simulink model "Mdl_Speed"  (R2024b)
settings: Solver=FixedStepDiscrete  StartTime=0.0  StopTime=10.0  FixedStep=0.1  RelTol=1e-3  EnableMultiTasking=on
values from neighbouring files (symbols this model uses):
  AI_TEMP_ADC_COUNT_1586 = mpt.Parameter    [Mdl_Speed_lookup.m]
  AI_TEMP_ADC_COUNT_1727 = mpt.Parameter    [Mdl_Speed_lookup.m]
  AI_TEMP_ADC_COUNT_1792 = mpt.Parameter    [Mdl_Speed_lookup.m]
  AI_TEMP_ADC_COUNT_1891 = mpt.Parameter    [Mdl_Speed_lookup.m]
  C_ADR = mpt.Parameter    [Mdl_Speed_lookup.m]
  C_CANADA = mpt.Parameter    [Mdl_Speed_lookup.m]
  C_EUROPE = mpt.Parameter    [Mdl_Speed_lookup.m]
  C_KOREA = mpt.Parameter    [Mdl_Speed_lookup.m]
  C_MEXICO = mpt.Parameter    [Mdl_Speed_lookup.m]
  C_UK = mpt.Parameter    [Mdl_Speed_lookup.m]
  C_USA = mpt.Parameter    [Mdl_Speed_lookup.m]
  eSP_ADR = mpt.Parameter    [Speed_Table_Type_param.m]
  eSP_CANADA = mpt.Parameter    [Speed_Table_Type_param.m]
  eSP_ECE = mpt.Parameter    [Speed_Table_Type_param.m]
  eSP_EUROPE = mpt.Parameter    [Speed_Table_Type_param.m]
  eSP_KOREA_FMVSS = mpt.Parameter    [Speed_Table_Type_param.m]
  eSP_KOREA_UN_R = mpt.Parameter    [Speed_Table_Type_param.m]
  eSP_MEXICO_FMVSS = mpt.Parameter    [Speed_Table_Type_param.m]
  eSP_MEXICO_UN_R = mpt.Parameter    [Speed_Table_Type_param.m]
  eSP_UK = mpt.Parameter    [Speed_Table_Type_param.m]
  eSP_USA = mpt.Parameter    [Speed_Table_Type_param.m]
  INDEX_MCUID0262 = mpt.Parameter    [Mdl_Speed_lookup.m]
  INDEX_MCUID0263 = mpt.Parameter    [Mdl_Speed_lookup.m]
  Initial_data = mpt.Parameter    [Mdl_Speed_lookup.m]
  MCUID0809 = mpt.Parameter    [Mdl_Speed_DD.m]
  MCUID0810 = mpt.Parameter    [Mdl_Speed_DD.m]
  MCUID_MAX_VAL = mpt.Parameter    [Mdl_Speed_lookup.m]
  MIN_SPEED_VALUE = mpt.Parameter    [Mdl_Speed_lookup.m]
  RESOLUTION_VAL_100 = mpt.Parameter    [Mdl_Speed_lookup.m]
  RESOLUTION_VAL_103 = mpt.Parameter    [Mdl_Speed_lookup.m]
  RESOLUTION_VAL_50 = mpt.Parameter    [Mdl_Speed_lookup.m]
  RESOLUTION_VAL_64 = mpt.Parameter    [Mdl_Speed_lookup.m]
  RESOLUTION_VAL_MINUS_100 = mpt.Parameter    [Mdl_Speed_lookup.m]
  SPEED_AVG_REF = mpt.Parameter    [Mdl_Speed_lookup.m]
  SPEED_CHECK_VALUE_ONE = mpt.Parameter    [Mdl_Speed_lookup.m]
  SPEED_UPDATE_0_28S = mpt.Parameter    [Mdl_Speed_lookup.m]
  SPEED_UPDATE_0_5S = mpt.Parameter    [Mdl_Speed_lookup.m]
  SPEED_UPDATE_1_5S = mpt.Parameter    [Mdl_Speed_lookup.m]
  SPEED_UPDATE_1S = mpt.Parameter    [Mdl_Speed_lookup.m]
  SPEED_ZERO = mpt.Parameter    [Mdl_Speed_lookup.m]
  VAL_ONE = mpt.Parameter    [Mdl_Speed_lookup.m]
  VAL_ZERO = mpt.Parameter    [Mdl_Speed_lookup.m]
undefined symbols (not defined in the file or in its folder): Arr_u8_100_type_instance, Arr_u8_1024_type_instance, Arr_u8_10_type_instance, Arr_u8_128_type_instance, Arr_u8_16_type_instance, Arr_u8_17_type_instance, Arr_u8_2048_type_instance, Arr_u8_256_type_instance, Arr_u8_32_type_instance, Arr_u8_3_type_instance, Arr_u8_46_type_instance, Arr_u8_48_type_instance, Arr_u8_61_type_instance, Arr_u8_64_type_instance, Arr_u8_8_type_instance, Arr_u8_9_type_instance, CLUSTER_ACTIVE, eIO_ADC_AI_TEMP_RTC, eSIGNAL_MISSING, eSIGNAL_NEVER_RECEIVED, eVehicleSpeedABSIn, IgnOff, IgnOn, IoHwAb_AdcSignalIdType_type_instance, IoHwAb_ErrorType_type_instance, pJustRcvdStatus, RxCan_SignalClearJustRcvdStatus, RxCan_SignalGetJustRcvdStatus, RxCan_SignalInvalidProcessingControl, RxCan_SignalMissingProcessingControl, RxCan_SignalNRProcessingControl, SignalId, SPEED_MAX_RESOLUTION, Status, tRxSignalId_type_instance, tRxSignalJustRcvdStatus_type_instance, tRxSignalStatus_type_instance
libraries: simulink x9
(part 3 of 3)

== system Mdl_Speed/Mdl_Speed_Task_sys/Digital_speed/Subsystem1/Interpolation&Trim_data/Subsystem/Speed_trimming_KM ==
  speed_avg : Inport  OutDataTypeStr=uint16
  Constant : Constant  Value=RESOLUTION_VAL_100  OutDataTypeStr=uint16
  Constant2 : Constant  Value=RESOLUTION_VAL_100
  Divide : Product  Inputs=*/  SaturateOnIntegerOverflow=on
  If : If  IfExpression=u1 < 50
  Merge : Merge
  Mod : Math  Operator=mod  SignedPower=on
  Speed_trim_Less_than_0.5 : Subsystem  TreatAsAtomicUnit=on
  Speed_trim_greater_than_equal_to_0.5 : Subsystem  TreatAsAtomicUnit=on
  Speed_trim : Outport  VectorParamsAs1DForOutWhenUnconnected=off
  wires:
  [Speed_avg] -> Divide/1
  Constant2/1 -> Divide/2
  If/1 -> Speed_trim_Less_than_0.5/Action
  Divide/1 -> Speed_trim_greater_than_equal_to_0.5/1(Speed_avg), Speed_trim_Less_than_0.5/1(Speed_avg)
  Speed_trim_Less_than_0.5/1(Speed_trim) -> Merge/1
  Speed_trim_greater_than_equal_to_0.5/1(Speed_trim) -> Merge/2
  If/2 -> Speed_trim_greater_than_equal_to_0.5/Action
  Mod/1 -> If/1
  [Speed_avg] -> Mod/1
  Constant/1 -> Mod/2
  Merge/1 -> Speed_trim/1
  speed_avg/1 -> [Speed_avg]

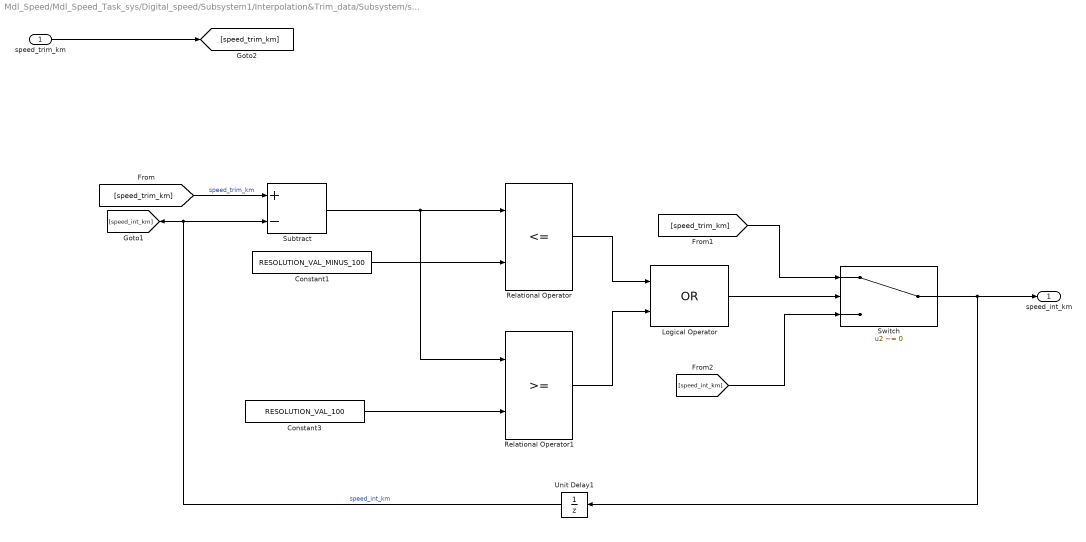
== system Mdl_Speed/Mdl_Speed_Task_sys/Digital_speed/Subsystem1/Interpolation&Trim_data/Subsystem/speed_internal_km ==
  speed_trim_km : Inport
  Constant1 : Constant  Value=RESOLUTION_VAL_MINUS_100  OutDataTypeStr=int8
  Constant3 : Constant  Value=RESOLUTION_VAL_100  OutDataTypeStr=uint16
  Logical Operator : Logic  Operator=OR  AllPortsSameDT=off  OutDataTypeStr=boolean
  Relational Operator : RelationalOperator  Operator=<=  OutDataTypeStr=boolean  RndMeth=Simplest  InputSameDT=off
  Relational Operator1 : RelationalOperator  OutDataTypeStr=boolean  RndMeth=Simplest  InputSameDT=off
  Subtract : Sum  Inputs=+-  OutDataTypeStr=int32
  Switch : Switch  Criteria=u2 ~= 0  SaturateOnIntegerOverflow=off  InputSameDT=off
  Unit Delay1 : UnitDelay  SampleTime=-1  StateName=Prev_speed_Int_km  HasFrameUpgradeWarning=on
  speed_int_km : Outport  VectorParamsAs1DForOutWhenUnconnected=off
  wires:
  [speed_trim_km] -> Subtract/1  "speed_trim_km"
  Unit Delay1/1 -> [speed_int_km], Subtract/2  "speed_int_km"
  Subtract/1 -> Relational Operator1/1, Relational Operator/1
  Constant1/1 -> Relational Operator/2
  Constant3/1 -> Relational Operator1/2
  Relational Operator/1 -> Logical Operator/1
  Relational Operator1/1 -> Logical Operator/2
  Logical Operator/1 -> Switch/2
  [speed_trim_km] -> Switch/1
  speed_trim_km/1 -> [speed_trim_km]
  Switch/1 -> speed_int_km/1, Unit Delay1/1
  [speed_int_km] -> Switch/3

== system Mdl_Speed/Mdl_Speed_Task_sys/Digital_speed/Subsystem1/Interpolation&Trim_data/Subsystem1/Speed_target_Miles ==
  Speed_int : Inport
  Constant2 : Constant  Value=RESOLUTION_VAL_100  OutDataTypeStr=uint16
  Constant3 : Constant  Value=RESOLUTION_VAL_100  OutDataTypeStr=uint16
  Divide : Product  Inputs=*/  SaturateOnIntegerOverflow=on
  If : If  IfExpression=u1 < 50
  If Action Subsystem : Subsystem  TreatAsAtomicUnit=on
  If Action Subsystem1 : Subsystem  TreatAsAtomicUnit=on
  Merge : Merge
  Mod : Math  Operator=mod  SignedPower=on
  speed_trg : Outport  VectorParamsAs1DForOutWhenUnconnected=off
  wires:
  Divide/1 -> If Action Subsystem1/1(In1), If Action Subsystem/1(In1)
  Constant3/1 -> Divide/2
  If/1 -> If Action Subsystem/Action
  [Speed_int] -> Divide/1
  If Action Subsystem1/1(Out1) -> Merge/2
  Merge/1 -> speed_trg/1
  [Speed_int] -> Mod/1
  Mod/1 -> If/1
  If/2 -> If Action Subsystem1/Action
  Constant2/1 -> Mod/2
  If Action Subsystem/1(Out1) -> Merge/1
  Speed_int/1 -> [Speed_int]

== system Mdl_Speed/Mdl_Speed_Task_sys/Digital_speed/Subsystem1/Interpolation&Trim_data/Subsystem1/Speed_trimming_Miles ==
  speed_avg : Inport  OutDataTypeStr=uint16
  Constant : Constant  Value=RESOLUTION_VAL_100  OutDataTypeStr=uint16
  Constant2 : Constant  Value=RESOLUTION_VAL_100
  Divide : Product  Inputs=*/  SaturateOnIntegerOverflow=on
  If : If  IfExpression=u1 < 50
  Merge : Merge
  Mod : Math  Operator=mod  SignedPower=on
  Speed_trim_Less_than_0.5 : Subsystem  TreatAsAtomicUnit=on
  Speed_trim_greater_than_equal_to_0.5 : Subsystem  TreatAsAtomicUnit=on
  Speed_trim : Outport  VectorParamsAs1DForOutWhenUnconnected=off
  wires:
  [Speed_avg] -> Divide/1
  Constant2/1 -> Divide/2
  If/1 -> Speed_trim_Less_than_0.5/Action
  Divide/1 -> Speed_trim_greater_than_equal_to_0.5/1(Speed_avg), Speed_trim_Less_than_0.5/1(Speed_avg)
  Speed_trim_Less_than_0.5/1(Speed_trim) -> Merge/1
  Speed_trim_greater_than_equal_to_0.5/1(Speed_trim) -> Merge/2
  If/2 -> Speed_trim_greater_than_equal_to_0.5/Action
  Mod/1 -> If/1
  [Speed_avg] -> Mod/1
  Constant/1 -> Mod/2
  Merge/1 -> Speed_trim/1
  speed_avg/1 -> [Speed_avg]

== system Mdl_Speed/Mdl_Speed_Task_sys/Digital_speed/Subsystem1/Interpolation&Trim_data/Subsystem1/kmtomiles_conversion1 ==
  Input : Inport  OutDataTypeStr=uint16
  Constant3 : Constant  Value=RESOLUTION_VAL_103
  Constant4 : Constant  Value=RESOLUTION_VAL_64
  Divide2 : Product  Inputs=**  OutDataTypeStr=uint32  RndMeth=Ceiling
  Divide3 : Product  Inputs=*/  OutDataTypeStr=uint16
  speed_avg : Outport  OutDataTypeStr=uint16  VectorParamsAs1DForOutWhenUnconnected=off
  wires:
  Divide2/1 -> Divide3/1
  Constant4/1 -> Divide2/2
  [speed_avg] -> Divide2/1
  Constant3/1 -> Divide3/2
  Divide3/1 -> speed_avg/1  "speed_avg"
  Input/1 -> [speed_avg]

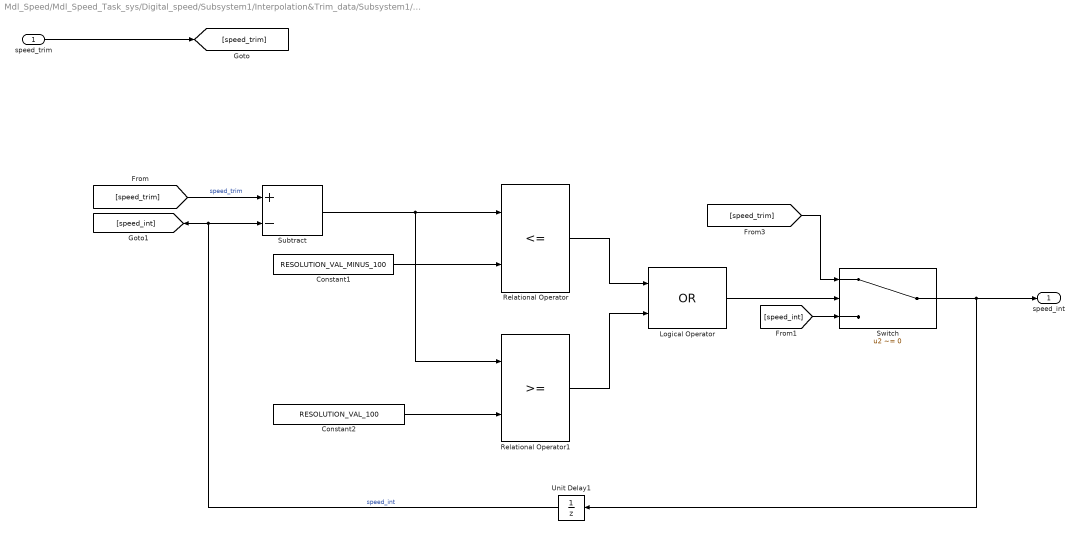
== system Mdl_Speed/Mdl_Speed_Task_sys/Digital_speed/Subsystem1/Interpolation&Trim_data/Subsystem1/speed_internal_Miles ==
  speed_trim : Inport
  Constant1 : Constant  Value=RESOLUTION_VAL_MINUS_100  OutDataTypeStr=int16
  Constant2 : Constant  Value=RESOLUTION_VAL_100  OutDataTypeStr=uint16
  Logical Operator : Logic  Operator=OR  AllPortsSameDT=off  OutDataTypeStr=boolean
  Relational Operator : RelationalOperator  Operator=<=  OutDataTypeStr=boolean  RndMeth=Simplest  InputSameDT=off
  Relational Operator1 : RelationalOperator  OutDataTypeStr=boolean  RndMeth=Simplest  InputSameDT=off
  Subtract : Sum  Inputs=+-  OutDataTypeStr=int16  AccumDataTypeStr=int32
  Switch : Switch  Criteria=u2 ~= 0  SaturateOnIntegerOverflow=off  InputSameDT=off
  Unit Delay1 : UnitDelay  SampleTime=-1  StateName=Prev_speed_Int  HasFrameUpgradeWarning=on
  speed_int : Outport  OutDataTypeStr=uint16  VectorParamsAs1DForOutWhenUnconnected=off
  wires:
  [speed_trim] -> Subtract/1  "speed_trim"
  Unit Delay1/1 -> [speed_int], Subtract/2  "speed_int"
  Subtract/1 -> Relational Operator1/1, Relational Operator/1
  Constant1/1 -> Relational Operator/2
  Constant2/1 -> Relational Operator1/2
  Relational Operator/1 -> Logical Operator/1
  Relational Operator1/1 -> Logical Operator/2
  Logical Operator/1 -> Switch/2
  [speed_trim] -> Switch/1
  speed_trim/1 -> [speed_trim]
  Switch/1 -> speed_int/1, Unit Delay1/1
  [speed_int] -> Switch/3

== system Mdl_Speed/Mdl_Speed_Task_sys/Digital_speed/Subsystem1/Interpolation&Trim_data/US_CAN_MAX/Subsystem ==
  Spd_Avg : Inport
  Constant4 : Constant  Value=SPEED_AVG_REF
  Data Store Read3 : DataStoreRead  DataStoreName=DSpeed_Int_Ref_US_CAN_MAX  IndexOptions=Index vector (dialog)  Indices=1  OutputSizes=1
  Lookup Table Dynamic : simulink/Lookup Tables/Lookup Table Dynamic  LookUpMeth=Interpolation-Use End Values  OutDataType=fixdt('uint16')  OutScaling=[]  OutputDataTypeScalingMode=Specify via dialog  OutDataTypeStr=uint16  RndMeth=Simplest  DoSatur=off
  Interpolated_Data : Outport  VectorParamsAs1DForOutWhenUnconnected=off
  wires:
  Spd_Avg/1 -> Lookup Table Dynamic/1
  Constant4/1 -> Lookup Table Dynamic/2
  Data Store Read3/1 -> Lookup Table Dynamic/3
  Lookup Table Dynamic/1 -> Interpolated_Data/1

== system Mdl_Speed/Mdl_Speed_Task_sys/Digital_speed/Subsystem1/Interpolation&Trim_data/Subsystem/Speed_target_km/If Action Subsystem ==
  In1 : Inport
  Action Port : ActionPort  ActionPortLabel=if(u1 < 50)
  Constant2 : Constant  Value=RESOLUTION_VAL_100  OutDataTypeStr=uint16
  Multiply : Product  OutDataTypeStr=uint16  SaturateOnIntegerOverflow=on
  Out1 : Outport  VectorParamsAs1DForOutWhenUnconnected=off
  wires:
  In1/1 -> Multiply/1
  Constant2/1 -> Multiply/2
  Multiply/1 -> Out1/1

== system Mdl_Speed/Mdl_Speed_Task_sys/Digital_speed/Subsystem1/Interpolation&Trim_data/Subsystem/Speed_target_km/If Action Subsystem1 ==
  In1 : Inport
  Action Port : ActionPort  ActionPortLabel=else
  Add : Sum  AccumDataTypeStr=uint16
  Constant1 : Constant  Value=VAL_ONE  OutDataTypeStr=uint16
  Constant2 : Constant  Value=RESOLUTION_VAL_100  OutDataTypeStr=uint16
  Multiply : Product  OutDataTypeStr=uint16  SaturateOnIntegerOverflow=on
  Out1 : Outport  VectorParamsAs1DForOutWhenUnconnected=off
  wires:
  Constant2/1 -> Multiply/2
  Constant1/1 -> Add/2
  In1/1 -> Add/1
  Add/1 -> Multiply/1
  Multiply/1 -> Out1/1

== system Mdl_Speed/Mdl_Speed_Task_sys/Digital_speed/Subsystem1/Interpolation&Trim_data/Subsystem/Speed_trimming_KM/Speed_trim_Less_than_0.5 ==
  Speed_avg : Inport
  Action Port : ActionPort  ActionPortLabel=if(u1 < 50)
  Constant2 : Constant  Value=RESOLUTION_VAL_100  OutDataTypeStr=uint16
  Multiply : Product  OutDataTypeStr=uint16
  Speed_trim : Outport  VectorParamsAs1DForOutWhenUnconnected=off
  wires:
  Speed_avg/1 -> Multiply/1
  Constant2/1 -> Multiply/2
  Multiply/1 -> Speed_trim/1

== system Mdl_Speed/Mdl_Speed_Task_sys/Digital_speed/Subsystem1/Interpolation&Trim_data/Subsystem/Speed_trimming_KM/Speed_trim_greater_than_equal_to_0.5 ==
  Speed_avg : Inport
  Action Port : ActionPort  ActionPortLabel=else
  Add : Sum  OutDataTypeStr=uint16  AccumDataTypeStr=uint16
  Constant1 : Constant  Value=RESOLUTION_VAL_50  OutDataTypeStr=uint16
  Constant2 : Constant  Value=RESOLUTION_VAL_100  OutDataTypeStr=uint16
  Multiply : Product
  Speed_trim : Outport  VectorParamsAs1DForOutWhenUnconnected=off
  wires:
  Multiply/1 -> Add/1
  Constant2/1 -> Multiply/2
  Speed_avg/1 -> Multiply/1
  Constant1/1 -> Add/2
  Add/1 -> Speed_trim/1

== system Mdl_Speed/Mdl_Speed_Task_sys/Digital_speed/Subsystem1/Interpolation&Trim_data/Subsystem1/Speed_target_Miles/If Action Subsystem ==
  In1 : Inport
  Action Port : ActionPort  ActionPortLabel=if(u1 < 50)
  Constant2 : Constant  Value=RESOLUTION_VAL_100  OutDataTypeStr=uint16
  Multiply : Product  OutDataTypeStr=uint16  SaturateOnIntegerOverflow=on
  Out1 : Outport  VectorParamsAs1DForOutWhenUnconnected=off
  wires:
  In1/1 -> Multiply/1
  Constant2/1 -> Multiply/2
  Multiply/1 -> Out1/1

== system Mdl_Speed/Mdl_Speed_Task_sys/Digital_speed/Subsystem1/Interpolation&Trim_data/Subsystem1/Speed_target_Miles/If Action Subsystem1 ==
  In1 : Inport
  Action Port : ActionPort  ActionPortLabel=else
  Add : Sum  AccumDataTypeStr=uint16
  Constant1 : Constant  Value=VAL_ONE  OutDataTypeStr=uint16
  Constant2 : Constant  Value=RESOLUTION_VAL_100  OutDataTypeStr=uint16
  Multiply : Product  OutDataTypeStr=uint16  SaturateOnIntegerOverflow=on
  Out1 : Outport  VectorParamsAs1DForOutWhenUnconnected=off
  wires:
  Constant2/1 -> Multiply/2
  Constant1/1 -> Add/2
  In1/1 -> Add/1
  Add/1 -> Multiply/1
  Multiply/1 -> Out1/1

== system Mdl_Speed/Mdl_Speed_Task_sys/Digital_speed/Subsystem1/Interpolation&Trim_data/Subsystem1/Speed_trimming_Miles/Speed_trim_Less_than_0.5 ==
  Speed_avg : Inport
  Action Port : ActionPort  ActionPortLabel=if(u1 < 50)
  Constant2 : Constant  Value=RESOLUTION_VAL_100  OutDataTypeStr=uint16
  Multiply : Product  OutDataTypeStr=uint16
  Speed_trim : Outport  VectorParamsAs1DForOutWhenUnconnected=off
  wires:
  Speed_avg/1 -> Multiply/1
  Constant2/1 -> Multiply/2
  Multiply/1 -> Speed_trim/1

== system Mdl_Speed/Mdl_Speed_Task_sys/Digital_speed/Subsystem1/Interpolation&Trim_data/Subsystem1/Speed_trimming_Miles/Speed_trim_greater_than_equal_to_0.5 ==
  Speed_avg : Inport
  Action Port : ActionPort  ActionPortLabel=else
  Add : Sum  OutDataTypeStr=uint16  AccumDataTypeStr=uint16
  Constant1 : Constant  Value=RESOLUTION_VAL_50  OutDataTypeStr=uint16
  Constant2 : Constant  Value=RESOLUTION_VAL_100  OutDataTypeStr=uint16
  Multiply : Product
  Speed_trim : Outport  VectorParamsAs1DForOutWhenUnconnected=off
  wires:
  Multiply/1 -> Add/1
  Constant2/1 -> Multiply/2
  Speed_avg/1 -> Multiply/1
  Constant1/1 -> Add/2
  Add/1 -> Speed_trim/1

== matlab function Mdl_Speed/Mdl_Speed_Task_sys/Digital_speed/Subsystem1/SpeedTable_Selection/Truth Table ==
  data: Country_code_func input; spd_selector output; MCUID_0809 input; MCUID_0810 input; C_USA parameter; C_CANADA parameter; C_MEXICO parameter; C_UK parameter; C_EUROPE parameter; C_KOREA parameter; C_ADR parameter; eSP_USA parameter; eSP_CANADA parameter; eSP_MEXICO_FMVSS parameter; eSP_MEXICO_UN_R parameter; eSP_UK parameter; eSP_EUROPE parameter; eSP_KOREA_FMVSS parameter; eSP_ADR parameter; eSP_ECE parameter; eSP_KOREA_UN_R parameter
function spd_selector = fcn(Country_code_func, MCUID_0809, MCUID_0810, C_USA, C_CANADA, C_MEXICO, C_UK, C_EUROPE, C_KOREA, C_ADR, eSP_USA, eSP_CANADA, eSP_MEXICO_FMVSS, eSP_MEXICO_UN_R, eSP_UK, eSP_EUROPE, eSP_KOREA_FMVSS, eSP_ADR, eSP_ECE, eSP_KOREA_UN_R)

aVarTruthTableCondition_1 = false;
aVarTruthTableCondition_2 = false;
aVarTruthTableCondition_3 = false;
aVarTruthTableCondition_4 = false;
aVarTruthTableCondition_5 = false;
aVarTruthTableCondition_6 = false;
aVarTruthTableCondition_7 = false;
aVarTruthTableCondition_8 = false;
aVarTruthTableCondition_9 = false;


% USA country Func

aVarTruthTableCondition_1 = logical((Country_code_func == C_USA));

% CANADA Country Func

aVarTruthTableCondition_2 = logical((Country_code_func == C_CANADA));

% Mexico with MCUID0809 =0

aVarTruthTableCondition_3 = logical(((Country_code_func == C_MEXICO) && (MCUID_0809 ==0)));

% Mexico with MCUID0809 =1

aVarTruthTableCondition_4 = logical(((Country_code_func == C_MEXICO) && (MCUID_0809 ==1)));

% UK country Func

aVarTruthTableCondition_5 = logical((Country_code_func == C_UK));

% EUR country Func

aVarTruthTableCondition_6 = logical((Country_code_func == C_EUROPE));

% Korea with MCUID0810 =0

aVarTruthTableCondition_7 = logical(((Country_code_func == C_KOREA) && (MCUID_0810 ==0)));

% Korea with MCUID0810 =1

aVarTruthTableCondition_8 = logical(((Country_code_func == C_KOREA) && (MCUID_0810 ==1)));

% Australia

aVarTruthTableCondition_9 = logical((Country_code_func == C_ADR));

if (aVarTruthTableCondition_1)
    aFcnTruthTableAction_1();
elseif (aVarTruthTableCondition_2)
    aFcnTruthTableAction_2();
elseif (aVarTruthTableCondition_3)
    aFcnTruthTableAction_3();
elseif (aVarTruthTableCondition_4)
    aFcnTruthTableAction_4();
elseif (aVarTruthTableCondition_5)
    aFcnTruthTableAction_5();
elseif (aVarTruthTableCondition_6)
    aFcnTruthTableAction_6();
elseif (aVarTruthTableCondition_7)
    aFcnTruthTableAction_7();
elseif (aVarTruthTableCondition_8)
    aFcnTruthTableAction_8();
elseif (aVarTruthTableCondition_9)
    aFcnTruthTableAction_9();
else % Default
    aFcnTruthTableAction_10();
end

function aFcnTruthTableAction_1()

% USA

spd_selector= eSP_USA;

function aFcnTruthTableAction_2()

% CANADA

spd_selector= eSP_CANADA;

function aFcnTruthTableAction_3()

% MEXICO_FMVSS

spd_selector= eSP_MEXICO_FMVSS;

function aFcnTruthTableAction_4()

% MEXICO_UN_R

spd_selector= eSP_MEXICO_UN_R;

function aFcnTruthTableAction_5()

% UK

spd_selector= eSP_UK;

function aFcnTruthTableAction_6()

% EUR

spd_selector= eSP_EUROPE;

function aFcnTruthTableAction_7()

% Korea_FMVSS

spd_selector= eSP_KOREA_FMVSS;

function aFcnTruthTableAction_8()

% Korea_UN-R

spd_selector= eSP_KOREA_UN_R;

function aFcnTruthTableAction_9()

% ADR

spd_selector= eSP_ADR;

function aFcnTruthTableAction_10()

% ECE

spd_selector= eSP_ECE;

== stateflow chart Mdl_Speed/Mdl_Speed_Task_sys/Digital_speed/Subsystem2/For Iterator Subsystem/If Action Subsystem/Chart ==
  (default) -> (junction 7) : {DSpeed_Int_Ref_Other[Index] =Initial_data[Index] }
  data: Initial_data input; Index input; DSpeed_Int_Ref_Other data_store_memory

== stateflow chart Mdl_Speed/Mdl_Speed_Task_sys/Digital_speed/Subsystem2/For Iterator Subsystem/If Action Subsystem1/Chart ==
  (default) -> (junction 7) : {DSpeed_Int_Ref_Other[Index] =DSpeed_Int_Ref_Other[Index] * SPEED_RESOLUTION }
  data: Index input; DSpeed_Int_Ref_Other data_store_memory; SPEED_RESOLUTION parameter

== stateflow chart Mdl_Speed/Mdl_Speed_Task_sys/Digital_speed/Subsystem2/For Iterator Subsystem/If Action Subsystem2/Chart ==
  (default) -> (junction 7) : {DSpeed_Int_Ref_US_CAN_MAX[Index] =Initial_data[Index] }
  data: Initial_data input; Index input; DSpeed_Int_Ref_US_CAN_MAX data_store_memory

== stateflow chart Mdl_Speed/Mdl_Speed_Task_sys/Digital_speed/Subsystem2/For Iterator Subsystem/If Action Subsystem3/Chart ==
  (default) -> (junction 7) : {DSpeed_Int_Ref_US_CAN_MAX[Index] =DSpeed_Int_Ref_US_CAN_MAX[Index] * SPEED_RESOLUTION }
  data: Index input; DSpeed_Int_Ref_US_CAN_MAX data_store_memory; SPEED_RESOLUTION parameter

== stateflow chart Mdl_Speed/Mdl_Speed_Task_sys/Digital_speed/Subsystem1/Chart3 ==
  (default) -> (junction 59) : {Index_x =0;Index_y =0;}
  (junction 59) -> (junction 32) [order 1] : [Index_x < SPEED_ARRAY_MAX_VALUE]
  (junction 33) -> (junction 59) [order 4]
  (junction 69) -> (junction 59) : {Index_x++;Index_y++;}
  (junction 59) -> (junction 31) [order 2]
  (junction 32) -> (junction 33) : {l_Speed_Array_Temp[Index_x][0] = data1[Index_y];
      | Index_x++;
      | }
  (junction 33) -> (junction 72) [order 1] : [Index_x == 1]{l_Speed_Array_Temp[Index_x][0] = data2}
  (junction 72) -> (junction 33)
  (junction 33) -> (junction 83) [order 2] : [Index_x == 3]{l_Speed_Array_Temp[Index_x][0] = 0}
  (junction 83) -> (junction 33)
  (junction 33) -> (junction 69) [order 3] : [(Index_x>3)&&(Index_x < SPEED_ARRAY_MAX_VALUE) ]
      | {l_Speed_Array_Temp[Index_x][0] = data[Index_y-2];}
  data: data input; data1 input; Index_y data_store_memory; l_Speed_Array_Temp output uint16 size=[22 2]; Index_x data_store_memory; SPEED_ARRAY_MAX_VALUE parameter; data2 input

== matlab function Mdl_Speed/Mdl_Speed_Task_sys/Digital_speed/Subsystem1/Speed_Update_Time_and_Avg_check/Speed_Update ==
  data: AI_TEMP input; Speed_update_time output; Spd_Table_selectn input; SPEED_CHECK_VALUE_ONE parameter; SPEED_UPDATE_0_28S parameter; SPEED_UPDATE_0_5S parameter; SPEED_UPDATE_1S parameter; SPEED_UPDATE_1_5S parameter; AI_TEMP_ADC_COUNT_1891 parameter; AI_TEMP_ADC_COUNT_1792 parameter; AI_TEMP_ADC_COUNT_1727 parameter; AI_TEMP_ADC_COUNT_1586 parameter; C_CANADA parameter; C_USA parameter; C_MEXICO parameter; eSP_KOREA_UN_R parameter; eSP_KOREA_FMVSS parameter; eSP_MEXICO_UN_R parameter; eSP_MEXICO_FMVSS parameter; eSP_USA parameter; eSP_CANADA parameter
function Speed_update_time = fcn(AI_TEMP, Spd_Table_selectn, SPEED_CHECK_VALUE_ONE, SPEED_UPDATE_0_28S, SPEED_UPDATE_0_5S, SPEED_UPDATE_1S, SPEED_UPDATE_1_5S, AI_TEMP_ADC_COUNT_1891, AI_TEMP_ADC_COUNT_1792, AI_TEMP_ADC_COUNT_1727, AI_TEMP_ADC_COUNT_1586, C_CANADA, C_USA, C_MEXICO, eSP_KOREA_UN_R, eSP_KOREA_FMVSS, eSP_MEXICO_UN_R, eSP_MEXICO_FMVSS, eSP_USA, eSP_CANADA)

aVarTruthTableCondition_1 = false;
aVarTruthTableCondition_2 = false;
aVarTruthTableCondition_3 = false;
aVarTruthTableCondition_4 = false;
aVarTruthTableCondition_5 = false;


% USA / CANADA / Mexico

aVarTruthTableCondition_1 = logical((Spd_Table_selectn == eSP_CANADA)|| (Spd_Table_selectn == eSP_USA)|| (Spd_Table_selectn == eSP_MEXICO_FMVSS)|| (Spd_Table_selectn == eSP_MEXICO_UN_R)|| (Spd_Table_selectn == eSP_KOREA_FMVSS)|| (Spd_Table_selectn == eSP_KOREA_UN_R));

% 0degC <= MCU temp

aVarTruthTableCondition_2 = logical((AI_TEMP >= AI_TEMP_ADC_COUNT_1891));

% -15degC <= MCU temp < 0degC

aVarTruthTableCondition_3 = logical((AI_TEMP >= AI_TEMP_ADC_COUNT_1792));

% -25degC <= MCU temp < -15degC

aVarTruthTableCondition_4 = logical((AI_TEMP >= AI_TEMP_ADC_COUNT_1727));

% MCU temp < -25degC

aVarTruthTableCondition_5 = logical((AI_TEMP >= AI_TEMP_ADC_COUNT_1586));

if (aVarTruthTableCondition_1)
    aFcnTruthTableAction_4();
elseif (aVarTruthTableCondition_2)
    aFcnTruthTableAction_4();
elseif (aVarTruthTableCondition_3)
    aFcnTruthTableAction_3();
elseif (aVarTruthTableCondition_4)
    aFcnTruthTableAction_2();
elseif (aVarTruthTableCondition_5)
    aFcnTruthTableAction_1();
else % Default
    aFcnTruthTableAction_4();
end

function aFcnTruthTableAction_1()

% Speed_update_time 1.5 S

Speed_update_time = SPEED_UPDATE_1_5S;

function aFcnTruthTableAction_2()

% Speed_update_time 1 S

Speed_update_time = SPEED_UPDATE_1S;

function aFcnTruthTableAction_3()

% Speed_update_time 0.5 S

Speed_update_time = SPEED_UPDATE_0_5S;

function aFcnTruthTableAction_4()

% Speed_update_time 0.28 S

Speed_update_time = SPEED_UPDATE_0_28S;
